simulink library "ESSLibrary"  (R2020a)
settings: Solver=VariableStepAuto  StartTime=0.0  StopTime=10.0  RelTol=1e-3
libraries: $bdroot x82, powerlib_meascontrol x10, simulink x7
(part 7 of 7)

== matlab function ESSLibrary/Dispatch/IfActionSubsystem/PrioritySelector/ReactivePowerPriority/ReactivePowerPriority_PQCurve/ReactivePowerEvaluator ==
  data: ReactivePowerCalc input; MaxQ_PQCurve input; ReactivePowerOut output; MinQ_PQCurve input; ECPAppPow input
function ReactivePowerOut = ReactivePowerEvaluator(ReactivePowerCalc, MaxQ_PQCurve, MinQ_PQCurve, ECPAppPow)
QPositiveLimit =0.0;
QNegativeLimit = 0.0;
if (ReactivePowerCalc >= 0.0)
    if (MaxQ_PQCurve >= ECPAppPow)
        QPositiveLimit = ECPAppPow;
    else
        QPositiveLimit = MaxQ_PQCurve;
    end
    if (ReactivePowerCalc >= QPositiveLimit)
        ReactivePowerOut = QPositiveLimit;
    else
        ReactivePowerOut = ReactivePowerCalc;
    end
else
    if (MinQ_PQCurve <=  (-1 *ECPAppPow))
        QNegativeLimit = (-1 *ECPAppPow);
    else
        QNegativeLimit = MinQ_PQCurve;
    end
    if (ReactivePowerCalc <= QNegativeLimit)
        ReactivePowerOut = QNegativeLimit;
    else
        ReactivePowerOut = ReactivePowerCalc;
    end
    
end

== matlab function ESSLibrary/Dispatch/IfActionSubsystem/PrioritySelector/ReactivePowerPriority/ReactivePowerPriority_PQCurve/QCapabilityCalculator/QMinCalculator ==
  data: X1 input; YMin output; Y1 input; X2 input; Y2 input; X3 input; Y3 input; X4 input; Y4 input; X5 input; Y5 input; X6 input; Y6 input; X7 input; Y7 input; X8 input; Y8 input; input input
function YMin     = fcn(X1,Y1,X2,Y2,X3,Y3,X4,Y4,X5,Y5,X6,Y6,X7,Y7,X8,Y8,input)

    XY = [X1 Y1 X2 Y2 X3 Y3 X4 Y4 X5 Y5 X6 Y6 X7 Y7 X8 Y8];

    [~,c] = size(PQ);

    YMin = 0;
    Y_negative = zeros(8,1);
    X_Ynegative = zeros(8,1);
    count = 1;
    for j = 2:2:c
        if XY(1,j) <=0
        Y_negative(count,1)= XY(1,j);
        X_Ynegative(count,1)= XY(1,j-1);
        count =count+1;
        end
    end

    if (count > 2)
        for i = 1:1:(count - 2)
            for j = i+1:1:(count-1)
                if(X_Ynegative(j,1) < X_Ynegative(i,1))
                    a=X_Ynegative(j,1);
                    X_Ynegative(j,1) = X_Ynegative(i,1);
                    X_Ynegative(i,1) = a;
                    a=Y_negative(j,1);
                    Y_negative(j,1) = Y_negative(i,1);
                    Y_negative(i,1) = a;
                end
            end
        end
        for i = 1 :1 : (count - 2)
           if ((input >= X_Ynegative(i,1)) && (input < X_Ynegative(i+1,1)))
               YMin = (((Y_negative(i+1,1)- Y_negative(i,1))/(X_Ynegative(i+1,1)- X_Ynegative(i,1)))* (input - X_Ynegative(i,1)))+ Y_negative(i,1);
           end
        end
    end
    if (input < X_Ynegative(1,1))
        YMin = Y_negative(1,1);
    end
    if (count > 1)
        if (input >= X_Ynegative(count-1,1))
            YMin = Y_negative(count-1);
        end
    end

end

== matlab function ESSLibrary/Dispatch/IfActionSubsystem/PrioritySelector/ReactivePowerPriority/ReactivePowerPriority_PQCurve/QCapabilityCalculator/YMaxCalculator ==
  data: X1 input; YMax output; Y1 input; X2 input; Y2 input; X3 input; Y3 input; X4 input; Y4 input; X5 input; Y5 input; X6 input; Y6 input; X7 input; Y7 input; X8 input; Y8 input; input input
function YMax      = fcn(X1,Y1,X2,Y2,X3,Y3,X4,Y4,X5,Y5,X6,Y6,X7,Y7,X8,Y8,input)

    XY = [X1 Y1 X2 Y2 X3 Y3 X4 Y4 X5 Y5 X6 Y6 X7 Y7 X8 Y8];

    [~,c] = size(PQ);

    YMax = 0;
    Y_positive = zeros(8,1);
    X_Ypositive= zeros(8,1);
    count = 1;

    for j = 2:2:c
        if XY(1,j) >=0
        Y_positive(count,1)= XY(1,j);
        X_Ypositive(count,1)= XY(1,j-1);
        count =count+1;
        end
    end

    if (count > 2)
        for i = 1:1:(count - 2)
            for j = i+1:1:(count-1)
                if(X_Ypositive(j,1) < X_Ypositive(i,1))
                    a=X_Ypositive(j,1);
                    X_Ypositive(j,1) = X_Ypositive(i,1);
                    X_Ypositive(i,1) = a;
                    a=Y_positive(j,1);
                    Y_positive(j,1) = Y_positive(i,1);
                    Y_positive(i,1) = a;
                end
            end
        end

        for i = 1 :1 : (count - 2)
           if ((input >= X_Ypositive(i,1)) && (input < X_Ypositive(i+1,1)))
               YMax = (((Y_positive(i+1,1)- Y_positive(i,1))/(X_Ypositive(i+1,1)- X_Ypositive(i,1)))* (input - X_Ypositive(i,1)))+ Y_positive(i,1);
               break;
           end
        end
    end
    if (input < X_Ypositive(1,1))
        YMax = Y_positive(1,1);
    end
    if (count > 1) 
        if (input >= X_Ypositive(count-1,1))
            YMax = Y_positive(count-1,1);
        end
    end

end

== matlab function ESSLibrary/DroopResponse_Points/If Action Subsystem/MATLAB Function1 ==
  data: ActVal input; Interpol output; Xdata input; Ydata input; ErrorCode output
function [Interpol, ErrorCode] = Droop(ActVal, Xdata, Ydata)
% mat= [Xdata;Ydata];
lx= length (Xdata);
% [~,c]= size(mat);
Interpol = 0;
ErrorCode = 0;

ly=length(Ydata);
if  lx~= ly
    Interpol = 0; 
    ErrorCode = 4;      % Number of variables in x-axis and y-axis are not same
end
if lx == ly
    for i = 1:1:lx-1
        if  Xdata(i) > Xdata(i+1)
            Interpol = 0; 
            ErrorCode = 5;      % Breakpoints are not in ascending order
        end
    if ActVal >= Xdata(i) && ActVal <= Xdata(i+1)     
        x1= Xdata(i);
        y1= Ydata(i);
        x2= Xdata(i+1);
        y2= Ydata(i+1);
        
        Interpol = y1 + (((ActVal-x1)*(y2-y1))/(x2-x1));     
    end 
    if ActVal < Xdata(1)
        Interpol = Ydata(1);
        ErrorCode = 2; % Actual value is less than the defined mimimum breakpoint
    end
    if ActVal > Xdata(lx)
        Interpol = Ydata(lx);
        ErrorCode = 3; % Actual value is greater than the defined max breakpoint
    end
    end

end
end

== matlab function ESSLibrary/Dispatch/IfActionSubsystem/RampLimiter1 ==
  data: Enable input; RampVal output; RefVal input; ActVal input; RampRateUp input; RampRateDn input; Reset input; RampEnd output; ErrorCode output
function [RampVal,RampEnd, ErrorCode]  = ramplimiter(Enable, RefVal, ActVal, RampRateUp, RampRateDn, Reset)
% ramplimiter is used to rampup or rampdown the actual value to reach the reference value. 
% Enable the function and provide the ramp rates to be applied on actual
% value, the function output the ramp value that gradually reached to the
% reference value.

% The reference value to be achieved by incresing or decreasing the actual
% value using the respective ramp rates, the actual value is basically a
% measurement. One the measured values reached the reference value, the
% funciton rasises an output rampend. If the reset input is raised then the 
% funciton outputs the measured value as it is. Here the reset input can be
% communication quality.

RampVal = 0;
RampEnd = false;
ErrorCode = 0;
if Enable ==1
    if (Reset == 0)
        RefRate = ((RefVal - ActVal));  
        if ((RefRate > 0)&& (RefRate >= RampRateUp))
            RampVal =  ActVal + RampRateUp;
            ErrorCode = 0;
       
        elseif ((RefRate < 0)&& (RefRate <= -RampRateDn))
            RampVal =   ActVal - RampRateDn;
            ErrorCode = 0;
            
        else
            RampEnd = true;
            RampVal = RefVal;
            ErrorCode = 0;
        end
    end
    if (Reset == 1)
        RampVal = ActVal; 
        ErrorCode = 0;
    end
end

if Enable == 0
    RampVal = ActVal; 
    RampEnd = true; 
    ErrorCode = 0;
end
end

== matlab function ESSLibrary/CoordinatedChDischMode/EnabledCoordinatedChDischMode/CrdChDischActivePowerEvaluator ==
  data: ActivePowerMeas input; Pout output; SoCMeas input; SoCTarget input; MaxChOrDischDuration input; TimeStep input; BattCapacity input; CrdChDischModeRampUp input; CrdChDischModeRampDown input; Tout output; ErrorCode output
function [Pout,Tout, ErrorCode] = CrdChDischActivePowerEvaluator(ActivePowerMeas,SoCMeas,SoCTarget,MaxChOrDischDuration,TimeStep,BattCapacity,CrdChDischModeRampUp,CrdChDischModeRampDown)
%This code calculates maximum possible Pref for Coordinadted charge discharge mode


%-------------------------
%MinChargingDuration1=t_constPreq+(Preq*((1/CrdChDischModeRampUp)+(1/CrdChDischModeRampDown))*TimeStep)-((ActivePowerMeas(1))*TimeStep/CrdChDischModeRampUp);
%EnergyOut1=(t_constPreq*Preq)+(Preq^2*((1/CrdChDischModeRampUp)+(1/CrdChDischModeRampDown))*TimeStep)-Preq*((ActivePowerMeas(1))*TimeStep/CrdChDischModeRampUp);
%ax2+bx+c=0 sloution
%-------------------------
persistent ChOrDischDuration;
if isempty(ChOrDischDuration)
    ChOrDischDuration=0;
end
ErrorCode = 0;
SocChange=abs((SoCTarget-SoCMeas)*3600/100*BattCapacity);
a=(-0.5*(TimeStep/CrdChDischModeRampUp)-0.5*(TimeStep/CrdChDischModeRampDown));
b= MaxChOrDischDuration-((ChOrDischDuration+1)*TimeStep)+((ActivePowerMeas * TimeStep)/CrdChDischModeRampUp);
c=(-0.5*ActivePowerMeas^2*(TimeStep/CrdChDischModeRampUp))+(0.5*ActivePowerMeas*TimeStep)-SocChange;

Preq1=(-b+sqrt(b^2-4*a*c))/(2*a);
disp(Preq1);
Preq2=(-b-sqrt(b^2-4*a*c))/(2*a);
%disp(Preq2);
t_constPreq1=MaxChOrDischDuration-Preq1*((TimeStep/CrdChDischModeRampUp)+(TimeStep/CrdChDischModeRampDown))+(ActivePowerMeas*(TimeStep/CrdChDischModeRampUp))-2*TimeStep;
%disp(t_constPreq1);
t_constPreq2=MaxChOrDischDuration-Preq2*((TimeStep/CrdChDischModeRampUp)+(TimeStep/CrdChDischModeRampDown))+(ActivePowerMeas*(TimeStep/CrdChDischModeRampUp))-2*TimeStep;
%disp(t_constPreq2);

if (t_constPreq1>0)
    Pout= Preq1;
    Tout=t_constPreq1;
elseif(t_constPreq2>0)
    Tout=t_constPreq2;
    Pout= Preq2;
else
    Pout=0;
    Tout=0; 
    ErrorCode = 030102;
end
ChOrDischDuration =ChOrDischDuration +1;
if ((ChOrDischDuration*TimeStep) > MaxChOrDischDuration)
    ChOrDischDuration=0;
end

== matlab function ESSLibrary/Dispatch/IfActionSubsystem/PrioritySelector/ReactivePowerPriority/ReactivePowerPriority_PQCurve/ActivePowerEvaluator1 ==
  data: ReactivePowerCalc input; ActivePowerOut output; ActivePowerCalc input; MaxP_PQCurve input; MinP_PQCurve input; ECPAppPow input; EnablePFLimit input; PFOperMax input; PFOperMin input
function ActivePowerOut = ActivePowerEvaluator(ReactivePowerCalc, ActivePowerCalc, MaxP_PQCurve, MinP_PQCurve, ECPAppPow, EnablePFLimit, PFOperMax, PFOperMin)
PPositiveLimit = 0.0;
PPositivePFLimit = 0.0;
PNegativeLimit = 0.0;
PNegativePFLimit = 0.0;
if (ActivePowerCalc >= 0.0)
    if (MaxP_PQCurve >= sqrt(power(ECPAppPow,2)- power(ReactivePowerCalc,2)))
        PPositiveLimit = sqrt(power(ECPAppPow,2)- power(ReactivePowerCalc,2));
    else
        PPositiveLimit = MaxP_PQCurve;
    end
    if (EnablePFLimit)
        if (ReactivePowerCalc >= 0.0)
            PPositivePFLimit = (ReactivePowerCalc*PFOperMax)/sqrt(1 - power(PFOperMax,2));
        else
            PPositivePFLimit = (ReactivePowerCalc*PFOperMin)/sqrt(1 - power(PFOperMin,2));
        end
    
        if (ActivePowerCalc >= min(PPositiveLimit, PPositivePFLimit))
            ActivePowerOut = min(PPositiveLimit, PPositivePFLimit);
        else
            ActivePowerOut = ActivePowerCalc;
        end
    else
        if (ActivePowerCalc >= PPositiveLimit)
            ActivePowerOut = PPositiveLimit;
        else
            ActivePowerOut = ActivePowerCalc;
        end
    end
    
else
    if (MinP_PQCurve <= (-1*sqrt(power(ECPAppPow,2)- power(ReactivePowerCalc,2))))
        PNegativeLimit = (-1*sqrt(power(ECPAppPow,2)- power(ReactivePowerCalc,2)));
    else
        PNegativeLimit = MaxP_PQCurve;
    end
    if (EnablePFLimit)
        if (ReactivePowerCalc >= 0.0)
            PNegativePFLimit = (ReactivePowerCalc*PFOperMin)/sqrt(1 - power(PFOperMin,2));
        else
            PNegativePFLimit = (ReactivePowerCalc*PFOperMax)/sqrt(1 - power(PFOperMax,2));
        end
    
        if (ActivePowerCalc <= max(PNegativeLimit, PNegativePFLimit))
            ActivePowerOut = max(PNegativeLimit, PNegativePFLimit);
        else
            ActivePowerOut = ActivePowerCalc;
        end
    else
        if (ActivePowerCalc <= PNegativeLimit)
            ActivePowerOut = PNegativeLimit;
        else
            ActivePowerOut = ActivePowerCalc;
        end
    end
    
end

== matlab function ESSLibrary/CoordinatedChDischMode/EnabledCoordinatedChDischMode/TimeTrigger ==
  settings: updateMethod=DISCRETE
  data: flag output; ActivePowerRequired input; ActivePowerOut output; TimeRequired input; ActivePowerMeas input; TimeStep input
function [flag,ActivePowerOut] = timetrigger(ActivePowerRequired,TimeRequired,ActivePowerMeas,TimeStep)
flag=0;
persistent TimeCount;
if isempty(TimeCount)
    TimeCount=0;
end
if (ActivePowerMeas >= ActivePowerRequired)
    flag=1;
    ActivePowerOut = ActivePowerRequired;
end

if ((TimeCount*TimeStep)>= TimeRequired)
    ActivePowerOut = 0.0;
    flag = 0;
end
if (flag==1)
    TimeCount=TimeCount+1;
   % disp(TimeCount);
else
    TimeCount=0;
end

== matlab function ESSLibrary/FixedPFMode/MATLAB Function ==
  data: PowerFactorSet input; ActivePowerMeasPU input; ReactivePowerOut output; ErrorCode output
function [ReactivePowerOut, ErrorCode] = ReactivePowerFromPowerFactor(PowerFactorSet, ActivePowerMeasPU)
ReactivePowerOut = 0.0;
ErrorCode = 0;
if ((PowerFactorSet > 0.0001)&&(PowerFactorSet < (-1*0.0001))) 
    if((1-power(PowerFactorSet,2))>0.0)
    ReactivePowerOut = (ActivePowerMeasPU/PowerFactorSet)*sqrt(1-power(PowerFactorSet,2));
    ErrorCode = 0;
    else
    ReactivePowerOut = 0.0;
    ErrorCode = 010102;
    end
else
    ReactivePowerOut = 0.0;
    ErrorCode = 010201;
end

== matlab function ESSLibrary/SoCManagement/IfActionSubsystem/RemainingEnergyCalculator ==
  data: ActivePowerMeasPU input; SoCFinal output; SoCMeas input; BatteryCapacity input; BasePower input; TimeStep input; ActivePowerRampUpRate input; ActivePowerRampDownRate input; SoCNextStep output
function [SoCFinal,SoCNextStep] = RemainingEnergyCalculator(ActivePowerMeasPU, SoCMeas, BatteryCapacity, BasePower ,TimeStep, ActivePowerRampUpRate,ActivePowerRampDownRate)
%disp('--------------Start-----------------');
NoOfRamps = 0;    % Number of ramps required to reach the measured active power

SoCFinal = 0;     % Final value of SoC that is calculated while active power ramps to zero vlaue

SoCNextStep = 0;  % SoC value that is calculated after the current execution

%Actual values of active power rampup and rampdown values in kW per time step
ActivePowerRampUpRate_kWPerTimeStep = ActivePowerRampUpRate*BasePower;
ActivePowerRampDownRate_kWPerTimeStep = ActivePowerRampDownRate*BasePower;
ActivePowerMeas = ActivePowerMeasPU*BasePower;

%SoCFinal and SoCNextStep calculations when BESS is discharging 
if (ActivePowerMeas >= 0)
   %calculating the nearest integer to the lower side of actual vlaue for number of ramps 
   NoOfRamps =  floor(ActivePowerMeas/ActivePowerRampUpRate_kWPerTimeStep);
%    disp('No Of Ramps');
%    disp(NoOfRamps);
   %Area under curve gives the energy required while active power ramps to zero
   AreaUnderCurve = (ActivePowerMeas*TimeStep*NoOfRamps)-(ActivePowerRampDownRate_kWPerTimeStep*TimeStep*0.5*NoOfRamps*(NoOfRamps-1));
%    disp('Area Under Curve');
%    disp(AreaUnderCurve);
   SoCFinal = ((SoCMeas*0.01*BatteryCapacity) - (AreaUnderCurve/3600))*(100/BatteryCapacity);% Measured SoC (in kWh)- Area under curve (in kWh); 1/3600 is the conversion ratio from kWs to kWh
%    disp('SoCFinal');
%    disp(SoCFinal);
   SoCNextStep = ((SoCMeas*0.01*BatteryCapacity) - ((ActivePowerMeas*TimeStep)/3600))*(100/BatteryCapacity);% Measured SoC (in kWh)- Area under  Active measured active power(in kWh); 1/3600 is the conversion ratio from kWs to kWh
%    disp('SoCNextStep');
%    disp(SoCNextStep); 
end

%SoCFinal and SoCNextStep calculations when BESS is charging 
if (ActivePowerMeas < 0)
   ActivePowerMeas = abs(ActivePowerMeas);
   %calculating the nearest integer to the lower side of actual vlaue for number of ramps
   NoOfRamps =  floor(ActivePowerMeas/ActivePowerRampUpRate_kWPerTimeStep); 
%    disp('No Of Ramps');
%    disp(NoOfRamps);
   %Area under curve gives the energy required while active power ramps to zero
   AreaUnderCurve = (ActivePowerMeas*TimeStep*NoOfRamps)-(ActivePowerRampUpRate_kWPerTimeStep*TimeStep*0.5*NoOfRamps*(NoOfRamps-1));
%    disp('Area Under Curve');
%    disp(AreaUnderCurve);
   SoCFinal = ((SoCMeas*0.01*BatteryCapacity) + (AreaUnderCurve/3600))*(100/BatteryCapacity);% Measured SoC (in kWh)- Area under curve (in kWh); 1/3600 is the conversion ratio from kWs to kWh
%    disp('SoCFinal');
%    disp(SoCFinal);
   SoCNextStep = ((SoCMeas*0.01*BatteryCapacity) + ((ActivePowerMeas*TimeStep)/3600))*(100/BatteryCapacity);% Measured SoC (in kWh)- Area under  Active measured active power(in kWh); 1/3600 is the conversion ratio from kWs to kWh
%    disp('SoCNextStep');
%    disp(SoCNextStep);  
end
% disp('--------------Stop-----------------');

== matlab function ESSLibrary/Disconnected/IfActionSubsystem/DisconnectedMode ==
  data: CBStatus input; ActivePowerOut output; ZeroActivePowerFlow input; ZeroReactivePowerFlow input; BreakerCmdTime input; ReactivePowerOut output; OpenCmd output; CloseCmd output; ErrorCode output; OpenTimeOut input; ResetDisconnected input
function [ActivePowerOut,ReactivePowerOut,OpenCmd, CloseCmd, ErrorCode] = DisconnectedMode(CBStatus, ZeroActivePowerFlow, ZeroReactivePowerFlow, BreakerCmdTime,OpenTimeOut, ResetDisconnected)
%--------------Initialization: Starts---------------
ActivePowerOut = 0.0;
ReactivePowerOut = 0.0;
CloseCmd = false;
OpenCmd = false;
ErrorCode = 0;
persistent prevOpenCmd TimeStepCounter OpenEnable ErrorCodeMeta;
if isempty(prevOpenCmd)  % Called the first time
    prevOpenCmd = false;      
end
if isempty(TimeStepCounter)  % Called the first time
    TimeStepCounter = 0;      
end
if isempty(OpenEnable)  % Called the first time
    OpenEnable = false;      
end
if isempty(ErrorCodeMeta)  % Called the first time
    ErrorCodeMeta = 0;      
end
%--------------Initialization: Ends---------------
%--------------Open Command assigning: starts-------
if ((prevOpenCmd == false)&& (OpenEnable == false))
    if ((CBStatus == 2) && ZeroActivePowerFlow && ZeroReactivePowerFlow)
        OpenEnable = true;
        ErrorCodeMeta = 0;
        OpenCmd = true;% If CBstatus detected close(2) and power flow is detected to be zero, the breaker is instructed to open
        TimeStepCounter = 1;%Time step is assigned  1st step counter
    end
end
TimeStepCounter = TimeStepCounter + 1;%Time step incremented in each execution cycle
if (prevOpenCmd == true)
    OpenCmd = true;% OpenCmd remains true till the 'BreakerCmdTime' is elapsed
    if (TimeStepCounter > BreakerCmdTime)% If 'BreakerCmdTime' is elapsed
        OpenCmd = false;
    end
end

if ((TimeStepCounter > OpenTimeOut) && (CBStatus == 2) && (OpenEnable == true))% If 'OpenTimeOut' is elapsed and CB status still under close condition
    TimeStepCounter = 0;
    ErrorCodeMeta = 010103;
end    
%--------------Open Command assigning: ends-------
prevOpenCmd = OpenCmd;
ErrorCode = ErrorCodeMeta;
%--------------Resettting the disconnected block:starts----------
if(ResetDisconnected == true)
 OpenEnable = false;
 ErrorCodeMeta = 0;
end

== matlab function ESSLibrary/MovAvgDeltaVoltCalc1/IfMovAvgFilter/DiscreteMovingAverage ==
  data: NoOfTS input; Out output; Inp input
function Out = fcn(NoOfTS,Inp)
% This code generates a moving average filter
NoOfTS = floor(NoOfTS);
Out = 0;
persistent buffer bufferIndex;
if isempty(buffer)  % Called the first time
    buffer = zeros(NoOfTS,1);
    bufferIndex = 0;  
    for i = 1:1:NoOfTS
    buffer(i)= Inp;
    end
end
bufferIndex         = bufferIndex + 1;
if bufferIndex == (NoOfTS+1)
    bufferIndex         =  1;
end
buffer(bufferIndex) = Inp;
for i = 1:1:NoOfTS
    Out = Out + buffer(i);
end
Out = Out/NoOfTS;
%disp("--------");

== matlab function ESSLibrary/Manual/IfActionSubsystem/MATLAB Function ==
  data: OpenCmdIn input; CloseCmdIn input; FreqWithinLimits input; VoltWithinLimits input; ActivePowerSetPU input; ReactivePoweSetPU input; ZeroActivePowerFlow input; ZeroReactivePowerFlow input; CBStatus input; ActivePowerOut output; BreakerCmdTime input; ReactivePowerOut output; OpenCmd output; CloseCmd output; ErrorCode output; OpenTimeOut input; CloseTimeOut input
function [ActivePowerOut,ReactivePowerOut,OpenCmd, CloseCmd, ErrorCode] = ManualMode(OpenCmdIn, CloseCmdIn, FreqWithinLimits, VoltWithinLimits, ActivePowerSetPU, ReactivePoweSetPU, ZeroActivePowerFlow, ZeroReactivePowerFlow, CBStatus, BreakerCmdTime, OpenTimeOut, CloseTimeOut)

%--------------Initialization: Starts---------------
ActivePowerOut = 0.0;
ReactivePowerOut = 0.0;
CloseCmd = false;
OpenCmd = false;
ErrorCode = 0;
persistent prevOpenCmd prevCloseCmd OpenEnable CloseEnable TimeStepCounter;
if isempty(prevOpenCmd)  % Called the first time
    prevOpenCmd = false;      
end
if isempty(prevCloseCmd)  % Called the first time
    prevCloseCmd = false;      
end
if isempty(OpenEnable)  % Called the first time
    OpenEnable = false;      
end
if isempty(CloseEnable)  % Called the first time
    CloseEnable = false;      
end
if isempty(TimeStepCounter)  % Called the first time
    TimeStepCounter = 0;      
end
%--------------Initialization: Ends-----------------

%--------------Open & Close input command prioritization: Starts---------
if (OpenCmdIn && ~prevOpenCmd)
    OpenEnable = true;
    CloseEnable = false;
end
if (CloseCmdIn && ~prevCloseCmd && ~OpenEnable)
   CloseEnable = true;
   OpenEnable = false;
end
%--------------Open & Close input command prioritization: Ends---------
%--------------Open Command assigning: starts--------------------------
if (OpenEnable)
    if ((CBStatus == 2) && ZeroActivePowerFlow && ZeroReactivePowerFlow)
        OpenCmd = true;% If CBstatus detected close(2) and power flow is detected to be zero, the breaker is instructed to open
        TimeStepCounter = 1;
    end
    if (prevOpenCmd == true)
        OpenCmd = true;% OpenCmd remains true till the 'BreakerCmdTime' is elapsed
        TimeStepCounter = TimeStepCounter + 1;%Time step incremented in each execution cycle
        if (TimeStepCounter > BreakerCmdTime)% If 'BreakerCmdTime' is elapsed
            OpenCmd = false;
        end
    end
    if ((TimeStepCounter > OpenTimeOut) && (CBStatus == 2))% If 'OpenTimeOut' is elapsed and CB status still under close condition
            OpenEnable = false;
            TimeStepCounter = 0;
            ErrorCode = 010103;
    end        
end
%--------------Open Command assigning: ends-----------------------------
%--------------Close Command assigning: starts--------------------------
if (CloseEnable)
    if ((CBStatus == 1) && FreqWithinLimits && VoltWithinLimits)
        CloseCmd = true;% If CBstatus detected open(1) and voltage and frequency is detected to be within limits
        TimeStepCounter = 1;
    end
    if (CBStatus == 2)% If CB status is detected close
        ActivePowerOut = ActivePowerSetPU;
        ReactivePowerOut = ReactivePoweSetPU;
    end
    if (prevCloseCmd == true)
        CloseCmd = true;% CloseCmd remains true till the 'BreakerCmdTime' is elapsed
        TimeStepCounter = TimeStepCounter + 1;%Time step incremented in each execution cycle
        if (TimeStepCounter > BreakerCmdTime)% If 'BreakerCmdTime' is elapsed
            CloseCmd = false;
        end
    end
    if ((TimeStepCounter > CloseTimeOut) && (CBStatus == 1))% If 'CloseTimeOut' is elapsed and CB status still under open condition
            TimeStepCounter = 0;
            ErrorCode = 020103;
    end
end
%--------------Close Command assigning: ends--------------------------
prevOpenCmd = OpenCmd;% Preserving the older value of open command
prevCloseCmd = CloseCmd;% Preserving the older value of open command
